simulink model "matlabpendulum"  (R2021a)
settings: Solver=FixedStepAuto  StartTime=0.0  StopTime=10  FixedStep=0.01  RelTol=1e-3
undefined symbols (not defined in the file): inits
libraries: vrlib x1
settings Model: EnablePacing=on  Creator=ASUS  LastModifiedBy=ASUS
settings DataIOCC: SaveFormat=Array  SaveOutput=off  SignalLogging=off  DSMLogging=off  SaveTime=off

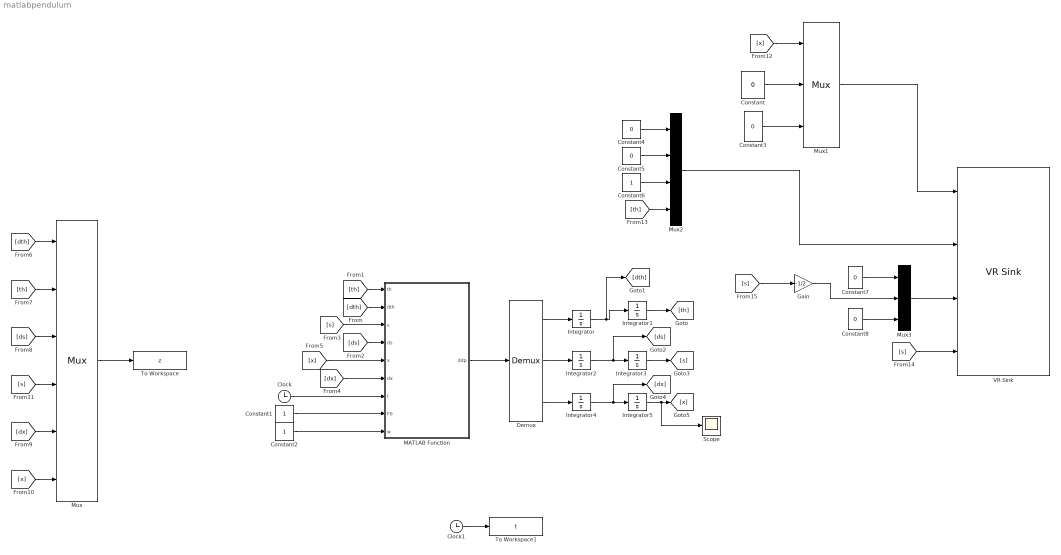
== system matlabpendulum ==
  Clock : Clock
  Clock1 : Clock
  Constant{,3..5,7..8} (6 alike) : Constant  Value=0
  Constant1 : Constant
  Constant2 : Constant
  Constant6 : Constant
  Demux : Demux  Outputs=3
  Gain : Gain  Gain=-1/2
  Integrator : Integrator  InitialCondition=inits(1)
  Integrator1 : Integrator  InitialCondition=deg2rad(inits(2))
  Integrator2 : Integrator  InitialCondition=inits(3)
  Integrator3 : Integrator  InitialCondition=inits(4)
  Integrator4 : Integrator  InitialCondition=inits(5)
  Integrator5 : Integrator  InitialCondition=inits(6)
  MATLAB Function : MATLAB Function  TreatAsAtomicUnit=on
  Mux : Mux  Inputs=6
  Mux1 : Mux  Inputs=3
  Mux2 : Mux
  Mux3 : Mux  Inputs=3
  Scope : Scope
  To Workspace : ToWorkspace  VariableName=z  SampleTime=-1
  To Workspace1 : ToWorkspace  VariableName=t  SampleTime=-1
  VR Sink : vrlib/VR Sink  InstantiateOnLoad=on  SampleTime=0.01  ViewEnable=on  RemoteChange=off  RemoteView=off  FieldsWritten=body1.translation.3.1.1.double#joint2.rotation.4.1.1.double#body2.translation.3.1.1.double#body2size.height.1.1.1.double  WorldFileName=vrr.wrl  AutoView=on  VideoDimensions=[]  AllowVariableSize=off
  wires:
  MATLAB Function/1(ddp) -> Demux/1
  Demux/1 -> Integrator/1
  Integrator/1 -> [dth], Integrator1/1
  Demux/2 -> Integrator2/1
  Integrator2/1 -> [ds], Integrator3/1
  Demux/3 -> Integrator4/1
  Integrator4/1 -> [dx], Integrator5/1
  Integrator1/1 -> [th]
  Integrator3/1 -> [s]
  Integrator5/1 -> Scope/1, [x]
  [dth] -> MATLAB Function/2(dth)
  [th] -> MATLAB Function/1(th)
  [ds] -> MATLAB Function/4(ds)
  [s] -> MATLAB Function/3(s)
  [dx] -> MATLAB Function/6(dx)
  [x] -> MATLAB Function/5(x)
  Constant1/1 -> MATLAB Function/8(F0)
  Constant2/1 -> MATLAB Function/9(w)
  Clock/1 -> MATLAB Function/7(t)
  [x] -> Mux/6
  [s] -> Mux/4
  [ds] -> Mux/3
  [th] -> Mux/2
  [dth] -> Mux/1
  [dx] -> Mux/5
  Mux/1 -> To Workspace/1
  Clock1/1 -> To Workspace1/1
  Constant/1 -> Mux1/2
  Constant3/1 -> Mux1/3
  [x] -> Mux1/1
  [th] -> Mux2/4
  Constant4/1 -> Mux2/1
  Constant5/1 -> Mux2/2
  Constant6/1 -> Mux2/3
  Mux1/1 -> VR Sink/1
  Mux2/1 -> VR Sink/2
  [s] -> VR Sink/4
  Constant7/1 -> Mux3/1
  Constant8/1 -> Mux3/3
  Mux3/1 -> VR Sink/3
  [s] -> Gain/1
  Gain/1 -> Mux3/2

== matlab function matlabpendulum/MATLAB Function ==
  data: th input; ddp output; dth input; s input; ds input; x input; dx input; t input; F0 input; w input
function ddp  = fcn(th,dth,s,ds,x,dx,t,F0,w)
M=5;
k=50;
l0=0.35;
m=0.3;
c=5;
g=9.81;
ddp=zeros(3,1);
%ddp(1)=ddth, (2)=dds, (3)=ddx
rho=(1/M)*(c*ds+k*(s-l0))*sin(th)+F0*M^-1*cos(w*t);
ddp(1,1)=(-1/s)*(2*dth*ds+rho*cos(th)+g*sin(th));
ddp(2,1)=(-c/m)*ds-(k/m)*(s-l0)+s*dth^2-rho*sin(th)+g*cos(th);
ddp(3,1)=rho;

end
